simulink library "G2ELib_V1"  (R2020b)
settings: Solver=VariableStepAuto  StartTime=0.0  StopTime=10.0  RelTol=1e-3
undefined symbols (not defined in the file or in its folder): ee_sli_rtmsupport, Filter, Filter_I_ini, Filter_V_ini, gcbh, GFM, GFM_L2, GFM_R2, Parameters_Ib, Parameters_Sb, Parameters_Un_dc, q_filter_wf, References_Q, References_Theta_Eg0, simlt, sps_rtmsupport, Vdc_loop
libraries: powerlib x48, simulink_extras x11, eeTransforms x10, pid_lib x8, spsSourcesModel x3, powerlib_meascontrol x3, spsVIMeasurementModel x3, spsFirstOrderFilterModel x3, spsSynchronousMachineModel x3, eeGeneralControl x2, eePowerMeasurement x1, sps3phSaturableTransformerModel x1
(part 2 of 5)

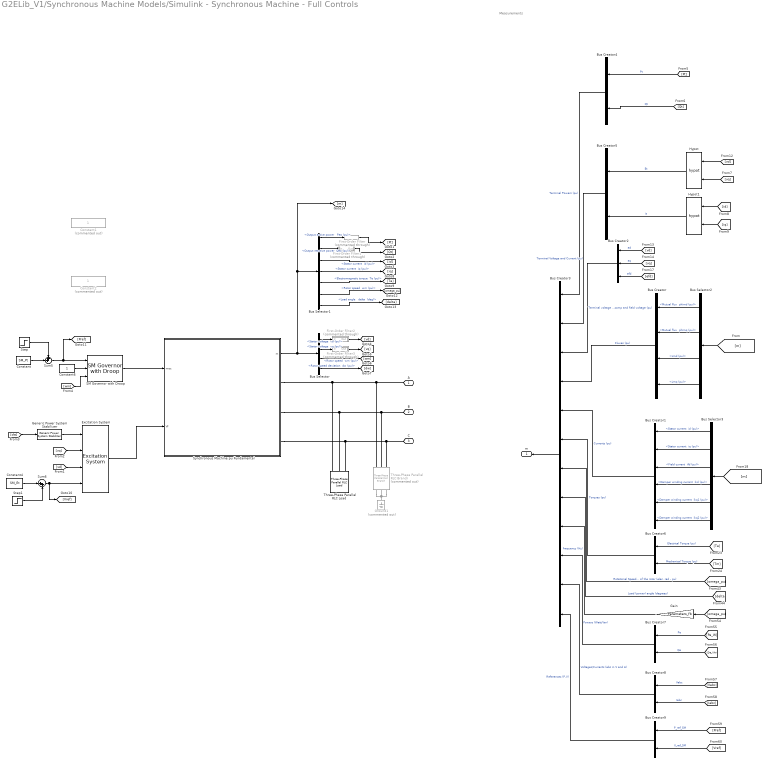
== system G2ELib_V1/Synchronous Machine Models/Simulink - Synchronous Machine - Full Controls ==
  note: Measurements
  Bus Creator : BusCreator  Inputs=4
  Bus Creator1 : BusCreator  Inputs=6
  Bus Creator2 : BusCreator  Inputs=3
  Bus Creator3 : BusCreator  Inputs=12
  Bus Creator{4..9} (6 alike) : BusCreator  Inputs=2
  Bus Selector : BusSelector  OutputSignals="dq0 components.Stator voltage  vd (pu),dq0 components.Stator voltage  vq (pu),Mechanical.Rotor speed  wm (pu),Mechanical.Rotor speed deviation  dw (pu)"
  Bus Selector1 : BusSelector  OutputSignals="Output active power   Peo (pu),Output reactive power  Qeo (pu),dq0 components.Stator current  id (pu),dq0 components.Stator current  iq (pu),Mechanical.Electromagnetic torque  Te (pu),Mechanical.Rotor speed  wm (pu),Load angle   delta  (deg)"
  Bus Selector2 : BusSelector  OutputSignals="dq0 components.Mutual flux  phimd (pu),dq0 components.Mutual flux  phimq (pu),dq0 components.Lmd (pu),dq0 components.Lmq (pu)"
  Bus Selector3 : BusSelector  OutputSignals="dq0 components.Stator current  id (pu),dq0 components.Stator current  iq (pu),dq0 components.Field current  ifd (pu),dq0 components.Damper winding current  ikd (pu),dq0 components.Damper winding current  ikq1 (pu),dq0 components.Damper winding current  ikq2 (pu)"
  Constant : Constant  Value=SM_Pt
  Constant1 : Constant  Commented=on
  Constant2 : Constant  Commented=on
  Constant4 : Constant  Value=SM_Et
  Constant6 : Constant
  Excitation System : sps_avr/Excitation System  tr=SM_Tr  reg=[ SM_Ka, SM_Ta ]  exc=[ SM_Ke, SM_Te ]  tgr=[ SM_Tb, SM_Tc ]  damp=[ SM_Kf, SM_Tf ]  sat=[ 0, 0 ]  lim=[ SM_Efmin, SM_Efmax, SM_Kp ]  v0=[SM_Et 1]
      settings: SourceProductBaseCode=PS
  First-Order Filter : powerlib_meascontrol/Filters/First-Order Filter  Commented=through  FilterType=Lowpass  Tc=20e-3  Ts=0  Initialize=on  Vac_Init=[0, 0, 60]  Vdc_Init=0  PlotResponse=off  FreqRange="[0,  200,  1]"
  First-Order Filter1 : Subsystem  Commented=through  DialogController=POWERSYS.PowerSysDialog  LoadFcn=sps_rtmsupport('LoadFcn', gcbh);  StartFcn=sps_rtmsupport('StartFcn', gcbh);  StopFcn=sps_rtmsupport('StopFcn', gcbh);  mask(First-Order Filter){FilterType=Lowpass, Tc=20e-3, Ts=0, Initialize=on, Vac_Init=[0, 0, 60], Vdc_Init=0, PlotResponse=off, FreqRange=[0,  200,  1]}
      mask prompts: FilterType "Filter type:"; Tc "Time constant (s):"; Ts "Sample time:"; Initialize "Initialize filter states"; Vac_Init "AC initial input [ Mag, Phase (degrees), Freq (Hz) ]:"; Vdc_Init "DC initial input:"; PlotResponse "Plot filter response"; FreqRange "Frequency range (Hz) [Start, End, Inc.]:"
      mask help:
      | Implement a first-order filter.
      |
      | Filter type = Lowpass -> H(s) =  1/(1+T.s)
      | Filter type = Highpass -> H(s) =  T.s/(1+T.s)
      mask init:
      | block=gcb;
      | [WantBlockChoice,Ts,sps] = powericon('FirstOrderFilterInit',block,FilterType,Tc,Initialize,Vac_Init,Vdc_Init,Ts);
      | powericon('FirstOrderFilterInit',FilterType, Tc, PlotResponse, FreqRange);
      | powericon('SetInternalModels','set',block,WantBlockChoice);
      settings: CopyFcn=sps_rtmsupport('CopyFcn', gcbh);  DeleteFcn=sps_rtmsupport('DeleteFcn', gcbh);  UndoDeleteFcn=sps_rtmsupport('UndoDeleteFcn', gcbh);  ModelCloseFcn=sps_rtmsupport('ModelCloseFcn', gcbh);  PreSaveFcn=sps_rtmsupport('PreSaveFcn', gcbh);  PostSaveFcn=sps_rtmsupport('PostSaveFcn', gcbh);  NameChangeFcn=sps_rtmsupport('NameChangeFcn', gcbh);  PreCopyFcn=sps_rtmsupport('PreCopyFcn', gcbh);  OpenFcn="sps_rtmsupport('OpenFcn', gcbh, [1  4  7]);"  CloseFcn=sps_rtmsupport('CloseFcn', gcbh);  PreDeleteFcn=sps_rtmsupport('PreDeleteFcn', gcbh);
      mask Help: helpview(psbhelp);
      mask TypeOptions FilterType: Lowpass | Highpass
      mask Callback Initialize: powericon('FirstOrderFilterInit',gcb);
      mask Callback PlotResponse: powericon('FirstOrderFilterInit',gcb);
      mask Display: plot(sps.X,sps.Y);
  First-Order Filter2 : Subsystem  Commented=through  DialogController=POWERSYS.PowerSysDialog  LoadFcn=sps_rtmsupport('LoadFcn', gcbh);  StartFcn=sps_rtmsupport('StartFcn', gcbh);  StopFcn=sps_rtmsupport('StopFcn', gcbh);  mask(First-Order Filter){FilterType=Lowpass, Tc=20e-3, Ts=0, Initialize=on, Vac_Init=[0, 0, 60], Vdc_Init=0, PlotResponse=off, FreqRange=[0,  200,  1]}
      mask prompts: FilterType "Filter type:"; Tc "Time constant (s):"; Ts "Sample time:"; Initialize "Initialize filter states"; Vac_Init "AC initial input [ Mag, Phase (degrees), Freq (Hz) ]:"; Vdc_Init "DC initial input:"; PlotResponse "Plot filter response"; FreqRange "Frequency range (Hz) [Start, End, Inc.]:"
      mask help:
      | Implement a first-order filter.
      |
      | Filter type = Lowpass -> H(s) =  1/(1+T.s)
      | Filter type = Highpass -> H(s) =  T.s/(1+T.s)
      mask init: same as G2ELib_V1/Synchronous Machine Models/Simulink - Synchronous Machine - Full Controls/First-Order Filter1
      settings: CopyFcn=sps_rtmsupport('CopyFcn', gcbh);  DeleteFcn=sps_rtmsupport('DeleteFcn', gcbh);  UndoDeleteFcn=sps_rtmsupport('UndoDeleteFcn', gcbh);  ModelCloseFcn=sps_rtmsupport('ModelCloseFcn', gcbh);  PreSaveFcn=sps_rtmsupport('PreSaveFcn', gcbh);  PostSaveFcn=sps_rtmsupport('PostSaveFcn', gcbh);  NameChangeFcn=sps_rtmsupport('NameChangeFcn', gcbh);  PreCopyFcn=sps_rtmsupport('PreCopyFcn', gcbh);  OpenFcn="sps_rtmsupport('OpenFcn', gcbh, [1  4  7]);"  CloseFcn=sps_rtmsupport('CloseFcn', gcbh);  PreDeleteFcn=sps_rtmsupport('PreDeleteFcn', gcbh);
      mask Help: helpview(psbhelp);
      mask TypeOptions FilterType: Lowpass | Highpass
      mask Callback Initialize: powericon('FirstOrderFilterInit',gcb);
      mask Callback PlotResponse: powericon('FirstOrderFilterInit',gcb);
      mask Display: plot(sps.X,sps.Y);
  First-Order Filter3 : Subsystem  Commented=through  DialogController=POWERSYS.PowerSysDialog  LoadFcn=sps_rtmsupport('LoadFcn', gcbh);  StartFcn=sps_rtmsupport('StartFcn', gcbh);  StopFcn=sps_rtmsupport('StopFcn', gcbh);  mask(First-Order Filter){FilterType=Lowpass, Tc=20e-3, Ts=0, Initialize=on, Vac_Init=[0, 0, 60], Vdc_Init=0, PlotResponse=off, FreqRange=[0,  200,  1]}
      mask prompts: FilterType "Filter type:"; Tc "Time constant (s):"; Ts "Sample time:"; Initialize "Initialize filter states"; Vac_Init "AC initial input [ Mag, Phase (degrees), Freq (Hz) ]:"; Vdc_Init "DC initial input:"; PlotResponse "Plot filter response"; FreqRange "Frequency range (Hz) [Start, End, Inc.]:"
      mask help:
      | Implement a first-order filter.
      |
      | Filter type = Lowpass -> H(s) =  1/(1+T.s)
      | Filter type = Highpass -> H(s) =  T.s/(1+T.s)
      mask init: same as G2ELib_V1/Synchronous Machine Models/Simulink - Synchronous Machine - Full Controls/First-Order Filter1
      settings: CopyFcn=sps_rtmsupport('CopyFcn', gcbh);  DeleteFcn=sps_rtmsupport('DeleteFcn', gcbh);  UndoDeleteFcn=sps_rtmsupport('UndoDeleteFcn', gcbh);  ModelCloseFcn=sps_rtmsupport('ModelCloseFcn', gcbh);  PreSaveFcn=sps_rtmsupport('PreSaveFcn', gcbh);  PostSaveFcn=sps_rtmsupport('PostSaveFcn', gcbh);  NameChangeFcn=sps_rtmsupport('NameChangeFcn', gcbh);  PreCopyFcn=sps_rtmsupport('PreCopyFcn', gcbh);  OpenFcn="sps_rtmsupport('OpenFcn', gcbh, [1  4  7]);"  CloseFcn=sps_rtmsupport('CloseFcn', gcbh);  PreDeleteFcn=sps_rtmsupport('PreDeleteFcn', gcbh);
      mask Help: helpview(psbhelp);
      mask TypeOptions FilterType: Lowpass | Highpass
      mask Callback Initialize: powericon('FirstOrderFilterInit',gcb);
      mask Callback PlotResponse: powericon('FirstOrderFilterInit',gcb);
      mask Display: plot(sps.X,sps.Y);
  Gain : Gain  Gain=Parameters_fb
  Generic Power System Stabilizer : powerlib/Machines/Generic Power System Stabilizer  Tsensor=SM_T_LP  K=SM_K_PSS  Twashout=SM_T_HP  Tleadlag1=[SM_T1n SM_T1d]  Tleadlag2=[SM_T2n SM_T2d]  VSlimits=[SM_VSmin SM_VSmax]  Vinit=0  Plot_On=off  MagdB_On=on  FreqRange=logspace(-2,2,500)
      settings: SourceProductBaseCode=PS
  Ground1 : powerlib/Elements/Ground  Commented=on  LConnTagsString=a
  Hypot : Math  Operator=hypot  SaturateOnIntegerOverflow=on
  Hypot1 : Math  Operator=hypot  SaturateOnIntegerOverflow=on
  SM Governor with Droop : eeSmGovernor/SM Governor with Droop  droop_percentage=SM_mp  T_G=SM_Tg  pu_throttle0=SM_Pt
      settings: SourceProductBaseCode=PS
  Step : Step  Time=T_Pref  After=delta_Pref  SampleTime=0
  Step1 : Step  Time=T_Vref  After=delta_Vref  SampleTime=0
  Sum5 : Sum  Inputs=++|
  Sum6 : Sum  Inputs=|++
  Synchronous Machine pu Fundamental : Subsystem  DialogController=POWERSYS.PowerSysDialog  LoadFcn=sps_rtmsupport('LoadFcn',gcbh);  StartFcn=sps_rtmsupport('StartFcn',gcbh);  StopFcn=sps_rtmsupport('StopFcn',gcbh);  mask(Synchronous Machine){PresetModel=No, MechanicalLoad=Mechanical power Pm, ShowDetailedParameters=on, RotorType=Round, Units=per unit fundamental parameters, MeasurementBus=off, NominalParameters=[ SM_Sn  SM_Un   Parameters_fb], Stator=[ SM_Ra  SM_Ll  SM_Lad  SM_Laq ], Field=[ SM_Rfd  SM_Lfd], Dampers2=[SM_R1d, SM_L1d, SM_R1q, SM_L1q, SM_R2q, SM_L2q ], Dampers1=[ 0.0284  0.1713  0.00619  0.7252 ], Mechanical=[ SM_H SM_K_D 1], PolePairs=20, InitialConditions=[0 ((SM_theta_0+SM_Phi)*180/pi) SM_It SM_It SM_It ((SM_alpha+SM_Phi)*180/pi) (-120+((SM_alpha+SM_Phi)*180/pi)) (120+((SM_Phi+SM_alpha)*180/pi)) 1], SetSaturation=off, Saturation=[0.6404,0.7127,0.8441,0.9214,0.9956,1.082,1.19,1.316,1.457;0.7,0.7698,0.8872,0.9466,0.9969,1.046,1.1,1.151,1.201], LoadFlowParameters=[1,0,0,0,0], TsPowergui=0, TsBlock=-1, IterativeModel=Trapezoidal non iterative, IterativeDiscreteModel=Trapezoidal non iterative, BusType=PV, Pref=SM_Pt*SM_Sn, Qref=0, Qmin=-inf, Qmax=inf, PLF=0, QLF=0}
      mask prompts: PresetModel "Preset  model:"; MechanicalLoad "Mechanical input:"; ShowDetailedParameters "Show detailed parameters"; RotorType "Rotor type:"; Units "Mask units:"; MeasurementBus "Use signal names to identify bus labels"; NominalParameters "Nominal power, line-to-line voltage and frequency [ Pn(VA)  Vn(Vrms)  fn(Hz) ]:"; Stator "Stator  [ Rs  Ll  Lmd  Lmq  (Lc) ] (pu):"; Field "Field  [ Rf  Llfd ] (pu):"; Dampers2 "Dampers  [ Rkd  Llkd  Rkq1  Llkq1  Rkq2  Llkq2 ] (pu):"; Dampers1 "Dampers  [ Rkd  Llkd  Rkq1  Llkq1 ] (pu):"; Mechanical "Inertia coefficient, friction factor, pole pairs [ H(s)  F(pu)  p() ]:"; PolePairs "Pole pairs p ():"; InitialConditions "Initial conditions [ dw(%)  th(deg)  ia,ib,ic(pu)  pha,phb,phc(deg)  Vf(pu) ]:"; SetSaturation "Simulate saturation"; Saturation "[ ifd; vt] (pu):"; LoadFlowParameters "Load Flow:   [Bus Type, Active Power,  UAB, phase of UAN ]"; TsPowergui "Sample time of powergui block:"; TsBlock "Sample time (-1 for inherited):"; IterativeDiscreteModel "Discrete solver model"; BusType "Generator type:"; Pref "Active power generation P (W):"; Qref "Reactive power generation Q (var):"; Qmin "Minimum reactive power Qmin (var):"; Qmax "Maximum reactive power Qmax (var):"; PLF "Load flow solution:  P_LF (W):"; QLF "Load flow solution:  Q_LF (var):"
      mask help: Implements a 3-phase synchronous machine modelled in the dq rotor reference frame. Stator windings are connected in wye to an internal neutral point.
      mask init:
      | block = gcb;
      | [Ts,SM,WantBlockChoice,X,Y] = powericon('SynchronousMachineInit',block,TsPowergui,TsBlock,MechanicalLoad,Units,RotorType,NominalParameters,Mechanical,PolePairs,InitialConditions,SetSaturation,Saturation,IterativeModel,MeasurementBus,Stator,Field,Dampers1,Dampers2);
      | powericon('SetInternalModels','set',block,WantBlockChoice); sps_rtmsupport('parametereditingmodes',block, [1 2 3 4 5 6 15 20 21 22]); 
      | powericon('ShaftInput',block);
      settings: CopyFcn=sps_rtmsupport('CopyFcn',gcbh); powericon('psbloadfunction',gcb,'gotofrom','UpdateGotoTag');  DeleteFcn=sps_rtmsupport('DeleteFcn',gcbh);  UndoDeleteFcn=sps_rtmsupport('UndoDeleteFcn',gcbh);  ModelCloseFcn=sps_rtmsupport('ModelCloseFcn',gcbh);  PreSaveFcn=sps_rtmsupport('PreSaveFcn',gcbh);  PostSaveFcn=sps_rtmsupport('PostSaveFcn',gcbh);  NameChangeFcn=sps_rtmsupport('NameChangeFcn',gcbh);  PreCopyFcn=sps_rtmsupport('PreCopyFcn',gcbh);  OpenFcn=sps_rtmsupport('OpenFcn',gcbh, [1 2 3 4 5 6 15 20 21 22]);  CloseFcn=sps_rtmsupport('CloseFcn',gcbh);  PreDeleteFcn=sps_rtmsupport('PreDeleteFcn',gcbh);
      mask Help: helpview(psbhelp);
      mask TypeOptions PresetModel: No | 01: 50Hz 400V 8.1kVA 1500RPM | 02: 50Hz 400V 16kVA 1500RPM | 03: 50Hz 400V 31.3kVA 1500RPM | 04: 50Hz 400V 42.5kVA 1500RPM | 05: 50Hz 400V 60kVA 1500RPM | 06: 50Hz 400V 85kVA 1500RPM | 07: 50Hz 400V 250kVA 1500RPM | 08: 50Hz 400V 325kVA 1500RPM | 09: 50Hz 400V 670kVA 1500RPM | 10: 50Hz 400V 910kVA 1500RPM | 11: 50Hz 400V 1320kVA 1500RPM | 12: 50Hz 400V 2000kVA 1500RPM | 13: 60Hz 460V 10.2kVA 1800RPM | 14: 60Hz 460V 20kVA 1800RPM | 15: 60Hz 460V 37.5kVA 1800RPM | 16: 60Hz 460V 52.5kVA 1800RPM | 17: 60Hz 460V 72.5kVA 1800RPM | 18: 60Hz 460V 100kVA 1800RPM | 19: 60Hz 460V 300kVA 1800RPM | 20: 60Hz 460V 406kVA 1800RPM | 21: 60Hz 460V 800kVA 1800RPM | 22: 60Hz 460V 1075kVA 1800RPM | 23: 60Hz 460V 1588kVA 1800RPM | 24: 60Hz 460V 2500kVA 1800RPM
      mask Callback PresetModel: powericon('SynchronousMachineCback',gcb,'per unit fundamental parameters');
      mask TypeOptions MechanicalLoad: Mechanical power Pm | Speed w | Mechanical rotational port
      mask Callback MechanicalLoad: powericon('SynchronousMachineCback',gcb,'per unit fundamental parameters');
      mask Callback ShowDetailedParameters: %powericon('SynchronousMachineCback',gcb,'per unit fundamental parameters');
      mask TypeOptions RotorType: Salient-pole | Round
      mask Callback RotorType: powericon('SynchronousMachineCback',gcb,'per unit fundamental parameters');
      mask TypeOptions Units: per unit fundamental parameters
      mask Callback SetSaturation: powericon('SynchronousMachineCback',gcb,'per unit fundamental parameters');
      mask TypeOptions IterativeModel: Trapezoidal non iterative | Trapezoidal iterative (alg. loop) | Forward Euler
      mask TypeOptions IterativeDiscreteModel: Trapezoidal non iterative | Trapezoidal iterative (alg. loop) | Trapezoidal robust | Backward Euler robust
      mask TypeOptions BusType: swing | PV | PQ
      mask Callback BusType: powericon('SynchronousMachineCback',gcb,'per unit fundamental parameters');
      mask Callback QLF: sps_rtmsupport('parametereditingmodes',gcbh, [1 2 3 4 5 6 15 20 21 22]);
      mask DialogControl Container4 Prompt: Configuration
      mask DialogControl Container9 Prompt: Measurement output
      mask DialogControl Container6 Prompt: Parameters
      mask DialogControl PlotSaturation Prompt: Plot
      mask DialogControl PlotSaturation Callback:
      | Saturation = evalin('base',get_param(gcbh,'Saturation'));
      | figure;plot(Saturation(1,:),Saturation(2,:),'*-');
      | xlabel(['ifd =', mat2str(Saturation(1,:),4)]);
      | ylabel(['vt =', mat2str(Saturation(2,:),4)]);
      mask DialogControl Advanced Prompt: Advanced
      mask DialogControl Note Prompt: Specialized Power Systems can automatically handle the advanced parameters of the block. For more information, see the settings in the 'Preferences' tab of Powergui block.
      mask DialogControl Control3 Prompt: Discrete solver model:
      mask DialogControl Control5 Prompt: This solver model is not recommended.
      mask DialogControl Control6 Prompt: Why?
      mask DialogControl Control6 Callback: web(fullfile(docroot, 'physmod/sps/powersys/ref/synchronousmachine.html#zmw57dd0e55004'))
      mask DialogControl Container7 Prompt: Load Flow
      mask Display:
      | plot(X.p1,Y.p1,X.p2,Y.p2,X.p3,Y.p3,X.p4,Y.p4,X.p5,Y.p5,X.p6,Y.p6,X.p7,Y.p7)
      | color('blue');
      | plot(X.p8,Y.p8)
      | plot(X.p9,Y.p9)
      | port_label('input',1,SM.PortLabel)
  Three-Phase Parallel RLC Branch : powerlib/Elements/Three-Phase Parallel RLC Branch  Commented=on  LConnTagsString=A|B|C  RConnTagsString=A|B|C  BranchType=R  Resistance=1e8  Inductance=1e-3  Capacitance=1e-11  Measurements=None
      settings: SourceProductBaseCode=PS
  Three-Phase Parallel RLC Load : powerlib/Elements/Three-Phase Parallel RLC Load  LConnTagsString=A|B|C  Configuration=Y (grounded)  NominalVoltage=SM_Un  Vabc=[1e3 1e3 1e3]  Vabcp=[1e3 1e3 1e3]  NominalFrequency=Parameters_fb  UnbalancedPower=off  ActivePower=100e3  InductivePower=0  CapacitivePower=0  Pabc=[10e3 9e3 11e3]  QLabc=[100 90 110]  QCabc=[100 90 110]  Pabcp=[10e3 9e3 11e3]  QLabcp=[100 90 110]  QCabcp=[100 90 110]  Measurements=None  LoadType=constant PQ
  A : PMIOPort  Side=Left
  B : PMIOPort  Port=2  Side=Left
  C : PMIOPort  Port=3  Side=Left
  m : Outport
  wires:
  Bus Creator9/1 -> Bus Creator3/12  "References (P,V)"
  [Vref] -> Bus Creator9/2  "V_ref_SM"
  [Pref] -> Bus Creator9/1  "P_ref_SM"
  Sum6/1 -> [Vref], Excitation System/1
  Step1/1 -> Sum6/2
  Constant4/1 -> Sum6/1
  Sum5/1 -> SM Governor with Droop/1, [Pref]
  Step/1 -> Sum5/1
  Constant/1 -> Sum5/2
  Hypot/1 -> Bus Creator5/1  "Et"
  [Qt] -> Bus Creator4/2  "Qt"
  [Pt] -> Bus Creator4/1  "Pt"
  Bus Creator3/1 -> m/1
  [Iabc] -> Bus Creator8/2  "Iabc"
  [Vabc] -> Bus Creator8/1  "Vabc"
  Bus Creator8/1 -> Bus Creator3/11  "Voltages/Currents (abc in V and A)"
  Bus Creator7/1 -> Bus Creator3/10  "Powers (Watt/Var)"
  [Qe_VAr] -> Bus Creator7/2  "Qe"
  [Pe_W] -> Bus Creator7/1  "Pe"
  Gain/1 -> Bus Creator3/9  "frequency (Hz)"
  [omega_pu] -> Gain/1
  [efd] -> Bus Creator2/3  "efd"
  [vq] -> Bus Creator2/2  "eq"
  [vd] -> Bus Creator2/1  "ed"
  [delta] -> Bus Creator3/8  "Load (power) angle (degrees)"
  [omega_pu] -> Bus Creator3/7  "Rotational Speed of the rotor (elec. rad - pu)"
  [Tm] -> Bus Creator6/2  "Mechanical Torque (pu)"
  Bus Creator6/1 -> Bus Creator3/6  "Torques (pu)"
  [Te] -> Bus Creator6/1  "Electrical Torque (pu)"
  Bus Creator1/1 -> Bus Creator3/5  "Currents (pu)"
  Bus Creator/1 -> Bus Creator3/4  "Fluxes (pu)"
  Bus Creator2/1 -> Bus Creator3/3  "Terminal voltage dq-comp and field voltage (pu)"
  Bus Creator5/1 -> Bus Creator3/2  "Terminal Voltage and Current (pu)"
  Bus Creator4/1 -> Bus Creator3/1  "Terminal Powers (pu)"
  [dw] -> Generic Power System Stabilizer/1
  [iq] -> Hypot1/2
  [id] -> Hypot1/1
  Constant6/1 -> SM Governor with Droop/2
  [vd] -> Excitation System/2
  Hypot1/1 -> Bus Creator5/2  "It"
  Bus Selector/1 -> First-Order Filter2/1(In)  "<Stator voltage  vd (pu)>"
  Bus Selector/4 -> [dw]  "<Rotor speed deviation  dw (pu)>"
  Bus Selector/3 -> [wm]  "<Rotor speed  wm (pu)>"
  Bus Selector/2 -> First-Order Filter3/1(In)  "<Stator voltage  vq (pu)>"
  Synchronous Machine pu Fundamental/1(m) -> [m], Bus Selector1/1, Bus Selector/1
  [vq] -> Excitation System/3
  [wm] -> SM Governor with Droop/3
  Bus Selector1/1 -> First-Order Filter/1  "<Output active power   Peo (pu)>"
  Bus Selector1/2 -> First-Order Filter1/1(In)  "<Output reactive power  Qeo (pu)>"
  [vq] -> Hypot/2
  [vd] -> Hypot/1
  Bus Selector1/3 -> [id]  "<Stator current  id (pu)>"
  Bus Selector1/4 -> [iq]  "<Stator current  iq (pu)>"
  Bus Selector1/5 -> [Te]  "<Electromagnetic torque  Te (pu)>"
  Bus Selector1/6 -> [omega_pu]  "<Rotor speed  wm (pu)>"
  Bus Selector1/7 -> [delta]  "<Load angle   delta  (deg)>"
  Generic Power System Stabilizer/1 -> Excitation System/4
  SM Governor with Droop/1 -> Synchronous Machine pu Fundamental/1(mec)
  Excitation System/1 -> Synchronous Machine pu Fundamental/2(Vf)
  First-Order Filter/1 -> [Pt]
  First-Order Filter1/1(Out) -> [Qt]
  First-Order Filter2/1(Out) -> [vd]
  First-Order Filter3/1(Out) -> [vq]
  [m] -> Bus Selector2/1
  Bus Selector2/1 -> Bus Creator/1  "<Mutual flux  phimd (pu)>"
  Bus Selector2/2 -> Bus Creator/2  "<Mutual flux  phimq (pu)>"
  [m] -> Bus Selector3/1
  Bus Selector3/1 -> Bus Creator1/1  "<Stator current  id (pu)>"
  Bus Selector3/2 -> Bus Creator1/2  "<Stator current  iq (pu)>"
  Bus Selector3/3 -> Bus Creator1/3  "<Field current  ifd (pu)>"
  Bus Selector3/4 -> Bus Creator1/4  "<Damper winding current  ikd (pu)>"
  Bus Selector3/5 -> Bus Creator1/5  "<Damper winding current  ikq1 (pu)>"
  Bus Selector3/6 -> Bus Creator1/6  "<Damper winding current  ikq2 (pu)>"
  Bus Selector2/3 -> Bus Creator/3  "<Lmd (pu)>"
  Bus Selector2/4 -> Bus Creator/4  "<Lmq (pu)>"
  connections:
  Synchronous Machine pu Fundamental/RConn1 -- Three-Phase Parallel RLC Branch/LConn1 -- A/RConn1 -- Three-Phase Parallel RLC Load/LConn1
  Synchronous Machine pu Fundamental/RConn2 -- B/RConn1 -- Three-Phase Parallel RLC Branch/LConn2 -- Three-Phase Parallel RLC Load/LConn2
  Synchronous Machine pu Fundamental/RConn3 -- Three-Phase Parallel RLC Load/LConn3 -- Three-Phase Parallel RLC Branch/LConn3 -- C/RConn1
  Ground1/LConn1 -- Three-Phase Parallel RLC Branch/RConn1 -- Three-Phase Parallel RLC Branch/RConn3 -- Three-Phase Parallel RLC Branch/RConn2

== system G2ELib_V1/DC//AC Converters/Voltage Source Converters (VSC)/Grid-Following VSC (GFL) ==
  note: Rename as "GFL_i" when you put in the network where "i" is the index of the GFL unit {1,2,...}
  note: Three phase voltage source for intialization and power flow - TO BE COMMENTED AFTER INITIALIZATION
  note: Proposed scope for GFL units
  Bus Selector2 : BusSelector  OutputSignals=P_GFL,Setpoints.P_set,Q_GFL,Setpoints.Q_Set,V_GFL,f_GFL,Vdc_GFL,Idc_GFL,I_GFL
  GFLi_measurements : Scope  NumInputPorts=7
  Init_GFL_i : Subsystem  DialogController=POWERSYS.PowerSysDialog  LoadFcn=sps_rtmsupport('LoadFcn',gcbh);  StartFcn=sps_rtmsupport('StartFcn',gcbh);  StopFcn=sps_rtmsupport('StopFcn',gcbh);  mask(Three-Phase Source){InternalConnection=Yg, VoltagePhases=off, Voltage=18000, PhaseAngle=2.1921, Voltage_phases=[25e3 25e3 25e3]/sqrt(3), PhaseAngles_phases=[0 -120 +120], Frequency=60, NonIdealSource=off, SpecifyImpedance=off, Resistance=0.8929, Inductance=16.58e-3, ShortCircuitLevel=100e6, BaseVoltage=18000, XRratio=7, BusType=PV, Pref=105000000, Qref=0, Prefabc=[10e3, 10e3, 10e3], Qrefabc=[0, 0, 0], Qmin=-inf, Qmax=inf}
      mask prompts: InternalConnection "Configuration:"; VoltagePhases "Specify internal voltages for each phase"; Voltage "Phase-to-phase voltage (Vrms):"; PhaseAngle "Phase angle of phase A (degrees):"; Voltage_phases "Line-to-neutral voltages [Va Vb Vc] (Vrms)"; PhaseAngles_phases "Phase angle of line-to-neutral voltages [phia phib phic] (deg)"; Frequency "Frequency (Hz):"; NonIdealSource "Internal"; SpecifyImpedance "Specify short-circuit level parameters"; Resistance "Source resistance (Ohms):"; Inductance "Source inductance (H):"; ShortCircuitLevel "3-phase short-circuit level at base voltage(VA):"; BaseVoltage "Base voltage (Vrms ph-ph):"; XRratio "X/R ratio:"; BusType "Generator type:"; Pref "Active power generation P (W)"; Qref "Reactive power generation Q (var)"; Prefabc "Active power generation [Pa Pb Pc] (W)"; Qrefabc "Reactive power generation [Qa Qb Qc] (var)"; Qmin "Minimum reactive power Qmin or [Qamin,Qbmin Qcmin] (var)"; Qmax "Maximum reactive power Qmax or [Qamax,Qbmax Qcmax] (var)"
      mask help: Three-phase voltage source in series with RL branch.
      mask init: same as G2ELib_V1/Miscellaneous Network Elements/Upstream Network
      settings: CopyFcn=sps_rtmsupport('CopyFcn',gcbh); powericon('psbloadfunction',gcb,'goto','UpdateGotoTag');  DeleteFcn=sps_rtmsupport('DeleteFcn',gcbh);  UndoDeleteFcn=sps_rtmsupport('UndoDeleteFcn',gcbh);  ModelCloseFcn=sps_rtmsupport('ModelCloseFcn',gcbh);  PreSaveFcn=sps_rtmsupport('PreSaveFcn',gcbh);  PostSaveFcn=sps_rtmsupport('PostSaveFcn',gcbh);  NameChangeFcn=sps_rtmsupport('NameChangeFcn',gcbh);  PreCopyFcn=sps_rtmsupport('PreCopyFcn',gcbh);  OpenFcn=sps_rtmsupport('OpenFcn',gcbh, [1,2,8,-9,15]);  CloseFcn=sps_rtmsupport('CloseFcn',gcbh);  PreDeleteFcn=sps_rtmsupport('PreDeleteFcn',gcbh);
      mask Help: helpview(psbhelp);
      mask TypeOptions InternalConnection: Y | Yn | Yg
      mask Callback InternalConnection: %powericon('ThreePhaseSourceCback',gcb);
      mask Callback VoltagePhases: powericon('ThreePhaseSourceCback',gcb);
      mask Callback NonIdealSource: powericon('ThreePhaseSourceCback',gcb);
      mask Callback SpecifyImpedance: powericon('ThreePhaseSourceCback',gcb);
      mask TypeOptions BusType: swing | PV | PQ
      mask Callback BusType: powericon('ThreePhaseSourceCback',gcb);
      mask Callback Qmax: sps_rtmsupport('parametereditingmodes',gcbh, [1,2,8,-9,15]);
      mask DialogControl Parameters Prompt: Parameters
      mask DialogControl Container7 Prompt: Source
      mask DialogControl Container6 Prompt: Impedance
      mask DialogControl LoadFlow Prompt: Load Flow
      mask Display:
      | plot(-180,-50,s5,50,s1,s2,s3,s4,[0,9,18,24,29,30,29,24,18,9,0,-9,-18,-24,-29,-30,-29,-24,-18,-9,0]*1.5-45, [30,29,24,18,9,0,-9,-18,-24,-29,-30,-29,-24,-18,-9,0,9,18,24,29,30]*0.8,[-150,-90],[0,0]);
      | plot(g1,g2,g3,g4,g5,g6);
      | plot([1 2 3 4 5 6 7 8 9 10 11 12 13 14 15 16 17 18 19 20 21].*2.5-72, [0,9,18,24,29,30,29,24,18,9,0,-9,-18,-24,-29,-30,-29,-24,-18,-9,0]./3)
  Mux2 : Mux  Inputs=2
  Mux6 : Mux  Inputs=2
  VSC - GFL - Ideal : Subsystem  mask{index_c=1, Parameters_fb=50, Parameters_wb=314.1593, GFL_Un=20000, GFL_Un_dc=32659.8632, GFL_Sn=1000000, GFL_Ib=40.8248, GFL_Ub=16329.9316, GFL_Ub_dc=32659.8632, GFL_Ib_dc=30.6186, GFL_Pref=0.5, GFL_Qref=0.1, GFL_V=1.0024, GFL_Theta_Eg0=0.0023037, GFL_Vdcref=32659.8632, Delta_Pref_GFL=0.1, Tsw_Pref_GFL=1.5, Delta_Qref_GFL=0.1, Tsw_Qref_GFL=2.5, GFL_DC_link_R=500000, GFL_DC_link_C=0.05, GFL_DC_link_Vdc_init=32659.8632, DC_link_Tdc=1e-3, GFL_R1_pu=0.0025, GFL_R2_pu=0.00013325, GFL_L1_pu=0.007854, GFL_L2_pu=0.00048, GFL_C_pu=0.10972, GFL_R1=1, GFL_R2=0.0533, GFL_L1=0.01, GFL_L2=0.00061115, GFL_C=8.731e-07, Controllers=PLL, GFL_Control_PLL=1, GFL_Control_VIM=0, GFL_Control_SU_theta=1, GFL_Control_SU_omega=1, GFL_vdc_Kp=-15999.9979, GFL_vdc_Ki=-2400725.019, GFL_KQ=-33.3333, GFL_Inner_current_loop_Kp=0.0725, GFL_Inner_current_loop_Ki=112.534, GFL_Inner_current_loop_Kffv=1, PLL_Kp=0.38197, PLL_Ki=22.9252, M_pll_0=-0.04362, VIM_wc=15.708, VIM_wc_ini=0, VIM_Iqd_sat=0.25, VIM_Rr_pu=0.0005, VIM_Lr_pu=0.05, VIM_Lm_pu=0.6, VIM_Rr=0.2, VIM_Lr=0.063662, VIM_Lm=0.76394, VIM_Kp=3.1416, VIM_Kd=0.001, VIM_Nd=100, VIM_H=5.04, VIM_J=0.00010213, VIM_D=0.8, VIM_Inertia_ini=0, VIM_Ke_ini=0, VIM_T_sync=0, VIM_f0=50, VIM_w0=1, GFL_Inner_current_loop_Int_ini_d=0.001247, GFL_Inner_current_loop_Int_ini_q=2.5553e-05, GFL_Filter_I_ini=[ 20.3591     -9.66764     -10.6914 ], GFL_Filter_V_ini=[ 16368.6462     -8063.31011     -8305.33605 ], GFL_Line_I_ini=[ 20.3974     -13.5751     -6.82233 ], GFL_Is0_dq0=[ 0.4988    0.010221           0 ], GFL_Eg0_dq0=[ 1.0024  4.3368e-19           0 ], GFL_Ig0_dq0=[ 0.4988    -0.09976           0 ], GFL_Vm0_dq0=[ 1.0036   0.0039431           0 ], M_d_0=-2.0777e-07, M_q_0=-0.00030664, GFL_theta=1.5793}
      mask prompts: index_c "Converter Number"; Parameters_fb "Nominal frequency (Hz)"; Parameters_wb "Nominal rotational frequency (rad/s)"; GFL_Un "Nominal AC voltage - Un (Urms)"; GFL_Un_dc "Nominal DC Voltage (V)"; GFL_Sn "Nominal Complex Power (VA)"; GFL_Ib "Base AC current (A)"; GFL_Ub "Base AC voltage (V)"; GFL_Ub_dc "Base DC voltage (V)"; GFL_Ib_dc "Base DC current (A)"; GFL_Pref "Active Power reference (p.u)"; GFL_Qref "Reactive Power reference (p.u)"; GFL_V "Initial Load Flow AC Voltage (p.u)"; GFL_Theta_Eg0 "Voltage angle (rad)"; GFL_Vdcref "DC voltage reference (V)"; Delta_Pref_GFL "Reference Active Power Steps"; Tsw_Pref_GFL "Time at which these steps take place (s)"; Delta_Qref_GFL "Reference Reactive Power Steps"; Tsw_Qref_GFL "Time at which these steps take place (s)"; GFL_DC_link_R "Parallel Resistance (ohm)"; GFL_DC_link_C "Parallel Capacitance (F)"; GFL_DC_link_Vdc_init "Initial Capacitor Voltage (V)"; DC_link_Tdc "DC-time response (s)"; GFL_R1_pu "F1 - Per unit Resistance"; GFL_R2_pu "F2 - Per unit Resistance"; GFL_L1_pu "F1 - Per unit Inductance"; GFL_L2_pu "F2 - Per unit Inductance"; GFL_C_pu "Per unit Capacitance"; GFL_R1 "F1 - Resistance (ohm)"; GFL_R2 "F2 - Resistance (ohm)"; GFL_L1 "F1 - Inductance (H)"; GFL_L2 "F2 - Inductance (H)"; GFL_C "Capacitance (C)"; Controllers "Select the control model"; GFL_Control_PLL "PLL"; GFL_Control_VIM "VIM"; GFL_Control_SU_theta "SU Theta (1:PLL, 2:VIM)"; GFL_Control_SU_omega "SU Omega (1:PLL, 2:VIM)"; GFL_vdc_Kp "Proportional constant - Kp"; GFL_vdc_Ki "Integral constant - Ki"; GFL_KQ "Integral constant - Ki"; GFL_Inner_current_loop_Kp "Proportional constant - Kp"; GFL_Inner_current_loop_Ki "Integral constant - Ki"; GFL_Inner_current_loop_Kffv "Feed-forward enable"; PLL_Kp "Proportional constant - Kp"; PLL_Ki "Integral constant - Ki"; M_pll_0 "Integral initialization"; VIM_wc "Filter cut-off frequency"; VIM_wc_ini "Filter initialization"; VIM_Iqd_sat "dq-current saturation"; VIM_Rr_pu "Per-unit rotor resistance"; VIM_Lr_pu "Per-unit rotor inductance"; VIM_Lm_pu "Per-unit mutual inductance"; VIM_Rr "Rotor resistance (ohm)"; VIM_Lr "Rotor inductance (H)"; VIM_Lm "Mutual inductance (H)"; VIM_Kp "Virtual Slip propotional action - Kp"; VIM_Kd "Virtual Slip derivative action - Kp"; VIM_Nd "Virtual Slip filter coefficient - Nd"; VIM_H "Inertia Constant (H)"; VIM_J "Equivalent moment of inertia (J)"; VIM_D "Damping (D)"; VIM_Inertia_ini "Inertia TF initialization"; VIM_Ke_ini "Electric Torque TF initialization"; VIM_T_sync "Synchronization Time (s)"; VIM_f0 "Initial rotor position (Hz)"; VIM_w0 "Initial rotor angular speed (rad/s)"; GFL_Inner_current_loop_Int_ini_d "d-axis"; GFL_Inner_current_loop_Int_ini_q "q-axis"; GFL_Filter_I_ini "Filter Current Init."; GFL_Filter_V_ini "Filter Voltage Init."; GFL_Line_I_ini "Line Current Init."; GFL_Is0_dq0 "Filter Current Init. (dq0)"; GFL_Eg0_dq0 "Filter Voltage Init. (dq0)"; GFL_Ig0_dq0 "Line Current Init. (dq0)"; GFL_Vm0_dq0 "Initial Voltage Modulation (dq0)"; M_d_0 "d-axis Vdc controller integrator"; M_q_0 "d-axis Qref controller integrator"; GFL_theta "Initial Phase (rad)"
      mask TypeOptions Controllers: PLL | VIM
      mask DialogControl DescTextVar Prompt: Voltage Source Converter modelled as 3-phase ideal voltage source with cascaded Grid-following/Feeding control topology
      mask DialogControl Container6 Prompt: General Parameters
      mask DialogControl Container9 Prompt: Index
      mask DialogControl Container10 Prompt: Nominal Values
      mask DialogControl Container54 Prompt: Base Values
      mask DialogControl Container12 Prompt: References
      mask DialogControl Container52 Prompt: Events
      mask DialogControl Container7 Prompt: Physical Model
      mask DialogControl Container13 Prompt: DC-Link
      mask DialogControl Container14 Prompt: Filter
      mask DialogControl Container8 Prompt: Control Selection
      mask DialogControl Container20 Prompt: Grid Angle Measurement
      mask DialogControl Container18 Prompt: Synchronization Unit Configuration and Selection
      mask DialogControl Container22 Prompt: Control Parameters
      mask DialogControl Container25 Prompt: Outer Loop Controllers
      mask DialogControl Container23 Prompt: D-axis Vdc Control
      mask DialogControl Container43 Prompt: Q-axis Qref Control
      mask DialogControl Container34 Prompt: Inner Loops
      mask DialogControl Container36 Prompt: Current Loop
      mask DialogControl Container46 Prompt: Grid Angle Measurement
      mask DialogControl Container47 Prompt: PLL
      mask DialogControl Container48 Prompt: VIM
      mask DialogControl Container40 Prompt: Initializations
      mask DialogControl Container41 Prompt: Inner Current Integrators
      mask DialogControl Container51 Prompt: Outer Loop Controls
      mask Display: image('$imagefile'); % Use "Edit Image" on toolstrip to change.
  wires:
  Mux6/1 -> GFLi_measurements/2  "Q_Q_ref"
  Bus Selector2/6 -> GFLi_measurements/4  "<f_GFL>"
  Bus Selector2/1 -> Mux2/1  "<P_GFL>"
  Bus Selector2/4 -> Mux6/2  "<Q_Set>"
  ? -> Bus Selector2/1
  Bus Selector2/8 -> GFLi_measurements/6  "<Idc_GFL>"
  Bus Selector2/5 -> GFLi_measurements/3  "<V_GFL>"
  Bus Selector2/7 -> GFLi_measurements/5  "<Vdc_GFL>"
  Bus Selector2/9 -> GFLi_measurements/7  "<I_GFL>"
  Bus Selector2/2 -> Mux2/2  "<P_set>"
  Mux2/1 -> GFLi_measurements/1  "P_P_ref"
  Bus Selector2/3 -> Mux6/1  "<Q_GFL>"
  VSC - GFL - Ideal/1(m) -> [GFLi_measurements]
  connections:
  Init_GFL_i/RConn1 -- VSC - GFL - Ideal/RConn1
  Init_GFL_i/RConn2 -- VSC - GFL - Ideal/RConn2
  Init_GFL_i/RConn3 -- VSC - GFL - Ideal/RConn3

== system G2ELib_V1/DC//AC Converters/Voltage Source Converters (VSC)/Grid-Forming VSC (GFM) ==
  note: Rename as "GFM_i" when you put in the network where "i" is the index of the GFM unit {1,2,...}
  note: Three phase voltage source for intialization and power flow - TO BE COMMENTED AFTER INITIALIZATION
  note: Proposed scope for GFM units
  Bus Selector13 : BusSelector  OutputSignals=P_GFM,Setpoints.P_set,Q_GFM,Setpoints.Q_set,V_GFM,Setpoints.Eg_set_d,f_GFM,I_GFM,Vdc_GFM,Idc_GFM
  GFMi_measurements : Scope  NumInputPorts=7
  Init_GFM_i : Subsystem  DialogController=POWERSYS.PowerSysDialog  LoadFcn=sps_rtmsupport('LoadFcn',gcbh);  StartFcn=sps_rtmsupport('StartFcn',gcbh);  StopFcn=sps_rtmsupport('StopFcn',gcbh);  mask(Three-Phase Source){InternalConnection=Yg, VoltagePhases=off, Voltage=18000, PhaseAngle=2.1921, Voltage_phases=[25e3 25e3 25e3]/sqrt(3), PhaseAngles_phases=[0 -120 +120], Frequency=60, NonIdealSource=off, SpecifyImpedance=off, Resistance=0.8929, Inductance=16.58e-3, ShortCircuitLevel=100e6, BaseVoltage=18000, XRratio=7, BusType=PV, Pref=105000000, Qref=0, Prefabc=[10e3, 10e3, 10e3], Qrefabc=[0, 0, 0], Qmin=-inf, Qmax=inf}
      mask prompts: InternalConnection "Configuration:"; VoltagePhases "Specify internal voltages for each phase"; Voltage "Phase-to-phase voltage (Vrms):"; PhaseAngle "Phase angle of phase A (degrees):"; Voltage_phases "Line-to-neutral voltages [Va Vb Vc] (Vrms)"; PhaseAngles_phases "Phase angle of line-to-neutral voltages [phia phib phic] (deg)"; Frequency "Frequency (Hz):"; NonIdealSource "Internal"; SpecifyImpedance "Specify short-circuit level parameters"; Resistance "Source resistance (Ohms):"; Inductance "Source inductance (H):"; ShortCircuitLevel "3-phase short-circuit level at base voltage(VA):"; BaseVoltage "Base voltage (Vrms ph-ph):"; XRratio "X/R ratio:"; BusType "Generator type:"; Pref "Active power generation P (W)"; Qref "Reactive power generation Q (var)"; Prefabc "Active power generation [Pa Pb Pc] (W)"; Qrefabc "Reactive power generation [Qa Qb Qc] (var)"; Qmin "Minimum reactive power Qmin or [Qamin,Qbmin Qcmin] (var)"; Qmax "Maximum reactive power Qmax or [Qamax,Qbmax Qcmax] (var)"
      mask help: Three-phase voltage source in series with RL branch.
      mask init: same as G2ELib_V1/Miscellaneous Network Elements/Upstream Network
      settings: CopyFcn=sps_rtmsupport('CopyFcn',gcbh); powericon('psbloadfunction',gcb,'goto','UpdateGotoTag');  DeleteFcn=sps_rtmsupport('DeleteFcn',gcbh);  UndoDeleteFcn=sps_rtmsupport('UndoDeleteFcn',gcbh);  ModelCloseFcn=sps_rtmsupport('ModelCloseFcn',gcbh);  PreSaveFcn=sps_rtmsupport('PreSaveFcn',gcbh);  PostSaveFcn=sps_rtmsupport('PostSaveFcn',gcbh);  NameChangeFcn=sps_rtmsupport('NameChangeFcn',gcbh);  PreCopyFcn=sps_rtmsupport('PreCopyFcn',gcbh);  OpenFcn=sps_rtmsupport('OpenFcn',gcbh, [1,2,8,-9,15]);  CloseFcn=sps_rtmsupport('CloseFcn',gcbh);  PreDeleteFcn=sps_rtmsupport('PreDeleteFcn',gcbh);
      mask Help: helpview(psbhelp);
      mask TypeOptions InternalConnection: Y | Yn | Yg
      mask Callback InternalConnection: %powericon('ThreePhaseSourceCback',gcb);
      mask Callback VoltagePhases: powericon('ThreePhaseSourceCback',gcb);
      mask Callback NonIdealSource: powericon('ThreePhaseSourceCback',gcb);
      mask Callback SpecifyImpedance: powericon('ThreePhaseSourceCback',gcb);
      mask TypeOptions BusType: swing | PV | PQ
      mask Callback BusType: powericon('ThreePhaseSourceCback',gcb);
      mask Callback Qmax: sps_rtmsupport('parametereditingmodes',gcbh, [1,2,8,-9,15]);
      mask DialogControl Parameters Prompt: Parameters
      mask DialogControl Container7 Prompt: Source
      mask DialogControl Container6 Prompt: Impedance
      mask DialogControl LoadFlow Prompt: Load Flow
      mask Display:
      | plot(-180,-50,s5,50,s1,s2,s3,s4,[0,9,18,24,29,30,29,24,18,9,0,-9,-18,-24,-29,-30,-29,-24,-18,-9,0]*1.5-45, [30,29,24,18,9,0,-9,-18,-24,-29,-30,-29,-24,-18,-9,0,9,18,24,29,30]*0.8,[-150,-90],[0,0]);
      | plot(g1,g2,g3,g4,g5,g6);
      | plot([1 2 3 4 5 6 7 8 9 10 11 12 13 14 15 16 17 18 19 20 21].*2.5-72, [0,9,18,24,29,30,29,24,18,9,0,-9,-18,-24,-29,-30,-29,-24,-18,-9,0]./3)
  Mux3 : Mux  Inputs=2
  Mux4 : Mux  Inputs=2
  Mux5 : Mux  Inputs=2
  VSC - GFM - Generic - Ideal : Subsystem  mask{index_c=1, Parameters_fb=50, Parameters_wb=2*pi*50, GFM_Un=20e3, GFM_Un_dc=2*20e3, GFM_Sn=5.22015e+07, GFM_Ib=2610.07662, GFM_Ub=20e3, GFM_Ub_dc=40e3, GFM_Ib_dc=562.5, GFM_Pref=0.5, GFM_Qref=0, GFM_Vref=1, GFM_Theta_Eg0=0, GFM_Vdcref=2*20e3, Delta_Pref_GFM=0, Tsw_Pref_GFM=0, Delta_Vref_GFM=0, Tsw_Vref_GFM=0, DC_link_R=500e6, DC_link_C=0.002, DC_link_Vdc_init=2*20e3, DC_link_Tdc=1e-3, GFM_R1_pu=0.005, GFM_R2_pu=0.15, GFM_L1_pu=0.066, GFM_L2_pu=0.038313, GFM_C_pu=0.066, GFM_R1=0.038313, GFM_R2=0.038313, GFM_L1=0.00365862, GFM_L2=0.00365862, GFM_C=2.741683e-05, Controllers=Droop, Control_PLL=0, Control_VIM=0, Control_MMU_QVDroop=1, Control_MMU_VSM=0, Control_dVOC=0, Control_MMU=1, Control_SU_PfDroop=1, Control_SU_Matching=0, Control_SU_VSM=0, Control_SU_theta=2, Control_SU_omega=2, Control_omega_set=3, Droop_mp=0.02, Droop_nq=0.0001, Droop_wc=0.1*2*pi*50, Droop_Int_ini=0, q_filter_wf=0.1*2*pi*50, q_filter_Int_ini=References_Q, p_filter_Int_ini=0.5, dVOC_eta=1*10/6, dVOC_alpha=12*6/10, Matching_K_theta=0.00005026, VSM_D=1e5, VSM_J=2e3, VSM_AVR_Kp=0.05, VSM_AVR_Ki=11.64, VSM_Dq=100, VSM_K=20, Vdc_loop_Ki=5, Vdc_loop_Kp=0.2, Vdc_loop_Kffi=0, Vdc_loop_Int_ini=2*20e3, Damping_resistor_Enable=1, Damping_resistor_Rv=0.09, Damping_resistor_W_RV=16.66, VI_Enable=0, VI_Rv_pu=0.001, VI_Lv_pu=0.1, TVI_K_RV=0.6716, TVI_Rho_XR=5, TVI_I_thresh_pu=1.2, Inner_voltage_loop_Kp=0.52, Inner_voltage_loop_Ki=1.161022, Inner_voltage_loop_Kffi=1, Inner_current_loop_Kp=0.738891, Inner_current_loop_Ki=1.19, Inner_current_loop_Kffv=1, PLL_Kp=0.4, PLL_Ki=4.69, PLL_Int_ini=0, VIM_wc=0.1*2*pi*50, VIM_wc_ini=0, VIM_Iqd_sat=0.25, VIM_Rr_pu=0.0005, VIM_Lr_pu=0.05, VIM_Lm_pu=0.6, VIM_Rr=0.0048, VIM_Lr=0.0015, VIM_Lm=0.0183, VIM_Kp=3.1416, VIM_Kd=0.001, VIM_Nd=100, VIM_H=0, VIM_J=0.0043, VIM_D=10, VIM_Inertia_ini=0, VIM_Ke_ini=0, VIM_T_sync=0.01, VIM_f0=50.08, VIM_w0=1.0016, SFR_Enable=1, SFR_Rc=0.001, SFR_dP_max=0.1, Inner_voltage_loop_Int_ini_d=0, Inner_voltage_loop_Int_ini_q=0, Inner_current_loop_Int_ini_d=0, Inner_current_loop_Int_ini_q=0, Damping_resistor_Int_ini=0.09, Filter_I_ini=[0 0 0], Filter_V_ini=[0 0 0], Line_I_ini=[0 0 0], Is0_dq0=[0 0 0], Eg0_dq0=[0 0 0], Ig0_dq0=[0 0 0], Vm0_dq0=[0 0 0], dVOC_ini_theta=0, dVOC_ini_R0=[1,0;0,1], Matching_Int_ini=0, GFM_theta=0}
      mask prompts: index_c "Converter Number"; Parameters_fb "Nominal frequency (Hz)"; Parameters_wb "Nominal rotational frequency (rad/s)"; GFM_Un "Nominal AC voltage - Un (Urms)"; GFM_Un_dc "Nominal DC Voltage (V)"; GFM_Sn "Nominal Complex Power (VA)"; GFM_Ib "Base AC current (A)"; GFM_Ub "Base AC voltage (V)"; GFM_Ub_dc "Base DC voltage (V)"; GFM_Ib_dc "Base DC current (A)"; GFM_Pref "Active Power reference (p.u)"; GFM_Qref "Reactive Power reference (p.u)"; GFM_Vref "AC Voltage reference (p.u)"; GFM_Theta_Eg0 "Voltage angle (rad)"; GFM_Vdcref "DC voltage reference (V)"; Delta_Pref_GFM "Reference Active Power Steps"; Tsw_Pref_GFM "Time at which these steps take place (s)"; Delta_Vref_GFM "Reference AC Voltage Steps"; Tsw_Vref_GFM "Time at which these steps take place (s)"; DC_link_R "Parallel Resistance (ohm)"; DC_link_C "Parallel Capacitance (F)"; DC_link_Vdc_init "Initial Capacitor Voltage (V)"; DC_link_Tdc "DC-Response time (s)"; GFM_R1_pu "F1 - Per unit Resistance"; GFM_R2_pu "F2 - Per unit Resistance"; GFM_L1_pu "F1 - Per unit Inductance"; GFM_L2_pu "F2 - Per unit Inductance"; GFM_C_pu "Per unit Capacitance"; GFM_R1 "F1 - Resistance (ohm)"; GFM_R2 "F2 - Resistance (ohm)"; GFM_L1 "F1 - Inductance (H)"; GFM_L2 "F2 - Inductance (H)"; GFM_C "Capacitance (C)"; Controllers "Select the control model"; Control_PLL "PLL"; Control_VIM "VIM"; Control_MMU_QVDroop "MMU - Q-V Droop"; Control_MMU_VSM "MMU - VSM"; Control_dVOC "MMU/SU dVOC"; Control_MMU "MMU (1:QV-droop, 2:dVOC, 3: no MMU,4: VSM AVR)"; Control_SU_PfDroop "SU - P-f Droop"; Control_SU_Matching "SU - Matching"; Control_SU_VSM "SU - VSM"; Control_SU_theta "SU Theta (1:dVOC, 2:Pf-droop, 3:Matching, 4:VSM)"; Control_SU_omega "SU Omega (1:dVOC, 2:Pf-droop, 3:Matching, 4:VSM)"; Control_omega_set "SU Omega Setpoint (1:PLL, 2:VIM, 3: 1 p.u)"; Droop_mp "P-f Droop (mp)"; Droop_nq "Q-V Droop (nq)"; Droop_wc "Second-order Droop filter cut-off frequency"; Droop_Int_ini "Second-order Droop filter initialization"; q_filter_wf "q-filter cut-off frequency"; q_filter_Int_ini "q-filter initialization"; p_filter_Int_ini "p-filter initialization"; dVOC_eta "Eta"; dVOC_alpha "Alpha"; Matching_K_theta "K_theta"; VSM_D "Damping"; VSM_J "Inertia"; VSM_AVR_Kp "AVR - Kp"; VSM_AVR_Ki "AVR - Ki"; VSM_Dq "Q-V proportional constant - Dq"; VSM_K "Q-V integral constant - K"; Vdc_loop_Ki "Integral constant - Ki"; Vdc_loop_Kp "Proportional constant - Kp"; Vdc_loop_Kffi "Feed-forward enable"; Vdc_loop_Int_ini "Integral initialization"; Damping_resistor_Enable "Enable the damping resistor"; Damping_resistor_Rv "Virtual Resistor (Rv)"; Damping_resistor_W_RV "Damping cut-off frequency"; VI_Enable "Enable the VI"; VI_Rv_pu "Virtual Resistor (p.u)"; VI_Lv_pu "Virtual Inductance (p.u)"; TVI_K_RV "TVI Resistor (K_Rv)"; TVI_Rho_XR "TVI R/X ratio (rho)"; TVI_I_thresh_pu "Threshold Current limit (p.u)"; Inner_voltage_loop_Kp "Proportional constant - Kp"; Inner_voltage_loop_Ki "Integral constant - Ki"; Inner_voltage_loop_Kffi "Feed-forward enable"; Inner_current_loop_Kp "Proportional constant - Kp"; Inner_current_loop_Ki "Integral constant - Ki"; Inner_current_loop_Kffv "Feed-forward enable"; PLL_Kp "Proportional constant - Kp"; PLL_Ki "Integral constant - Ki"; PLL_Int_ini "Integral initialization"; VIM_wc "Filter cut-off frequency"; VIM_wc_ini "Filter initialization"; VIM_Iqd_sat "dq-current saturation"; VIM_Rr_pu "Per-unit rotor resistance"; VIM_Lr_pu "Per-unit rotor inductance"; VIM_Lm_pu "Per-unit mutual inductance"; VIM_Rr "Rotor resistance (ohm)"; VIM_Lr "Rotor inductance (H)"; VIM_Lm "Mutual inductance (H)"; VIM_Kp "Virtual Slip propotional action - Kp"; VIM_Kd "Virtual Slip derivative action - Kp"; VIM_Nd "Virtual Slip filter coefficient - Nd"; VIM_H "Inertia Constant (H)"; VIM_J "Equivalent moment of inertia (J)"; VIM_D "Damping (D)"; VIM_Inertia_ini "Inertia TF initialization"; VIM_Ke_ini "Electric Torque TF initialization"; VIM_T_sync "Synchronization Time (s)"; VIM_f0 "Initial rotor position (Hz)"; VIM_w0 "Initial rotor angular speed (rad/s)"; SFR_Enable "Enable/Disable"; SFR_Rc "SFR Constant"; SFR_dP_max "Maximum Regulation (p.u)"; Inner_voltage_loop_Int_ini_d "d-axis"; Inner_voltage_loop_Int_ini_q "q-axis"; Inner_current_loop_Int_ini_d "d-axis"; Inner_current_loop_Int_ini_q "q-axis"; Damping_resistor_Int_ini "Damping resistor integrator"; Filter_I_ini "Filter Current Init."; Filter_V_ini "Filter Voltage Init."; Line_I_ini "Line Current Init."; Is0_dq0 "Filter Current Init. (dq0)"; Eg0_dq0 "Filter Voltage Init. (dq0)"; Ig0_dq0 "Line Current Init. (dq0)"; Vm0_dq0 "Initial Voltage Modulation (dq0)"; dVOC_ini_theta "dVOC Initial Theta"; dVOC_ini_R0 "dVOC R(Kappa) initial"; Matching_Int_ini "Matching integral initialization"; GFM_theta "Initial Phase (rad)"
      mask TypeOptions Controllers: Droop | Droop+PLL | Droop+VIM | dVOC | Matching | VSM
      mask DialogControl Container6 Prompt: General Parameters
      mask DialogControl Container9 Prompt: Index
      mask DialogControl Container10 Prompt: Nominal Values
      mask DialogControl Container54 Prompt: Base Values
      mask DialogControl Container12 Prompt: References
      mask DialogControl Container52 Prompt: Events
      mask DialogControl Container7 Prompt: Physical Model
      mask DialogControl Container13 Prompt: DC-Link
      mask DialogControl Container14 Prompt: Filter
      mask DialogControl Container8 Prompt: Control Selection
      mask DialogControl Container20 Prompt: Grid Angle Measurement
      mask DialogControl Container21 Prompt: Magnitude Modulation Control Configuration and Selection
      mask DialogControl Container18 Prompt: Synchronization Unit Configuration and Selection
      mask DialogControl Container22 Prompt: Control Parameters
      mask DialogControl Container25 Prompt: Outer Loop Controllers
      mask DialogControl Container23 Prompt: GFM-Droop
      mask DialogControl Container24 Prompt: Filters
      mask DialogControl Container43 Prompt: dVOC
      mask DialogControl Container44 Prompt: Matching
      mask DialogControl Container45 Prompt: VSM
      mask DialogControl Container26 Prompt: DC-Side Controller
      mask DialogControl Container27 Prompt: Tertiary Functions
      mask DialogControl Container28 Prompt: Damping Resistor
      mask DialogControl Container31 Prompt: Virtual Impedance (VI)
      mask DialogControl Container33 Prompt: Transient Virtual Impedance (TVI)
      mask DialogControl Container34 Prompt: Inner Loops
      mask DialogControl Container35 Prompt: Voltage Loop
      mask DialogControl Container36 Prompt: Current Loop
      mask DialogControl Container46 Prompt: Grid Angle Measurement
      mask DialogControl Container47 Prompt: PLL
      mask DialogControl Container48 Prompt: VIM
      mask DialogControl Container37 Prompt: Secondary Frequency Regulation
      mask DialogControl Container40 Prompt: Initializations
      mask DialogControl container42 Prompt: Inner Voltage Integrators
      mask DialogControl Container41 Prompt: Inner Current Integrators
      mask DialogControl Container51 Prompt: Outer Loop Controls
      mask Display: image('$imagefile'); % Use "Edit Image" on toolstrip to change.
  wires:
  Bus Selector13/6 -> Mux4/2  "<Eg_set_d>"
  Bus Selector13/9 -> GFMi_measurements/6  "<Vdc_GFM>"
  Bus Selector13/3 -> Mux5/1  "<Q_GFM>"
  Bus Selector13/8 -> GFMi_measurements/5  "<I_GFM>"
  Bus Selector13/10 -> GFMi_measurements/7  "<Idc_GFM>"
  Bus Selector13/2 -> Mux3/2  "<P_set>"
  Mux5/1 -> GFMi_measurements/2  "Q_Q_ref"
  ? -> Bus Selector13/1
  Bus Selector13/1 -> Mux3/1  "<P_GFM>"
  Mux3/1 -> GFMi_measurements/1  "P_P_ref"
  Bus Selector13/7 -> GFMi_measurements/4  "<f_GFM>"
  Bus Selector13/4 -> Mux5/2  "<Q_set>"
  Bus Selector13/5 -> Mux4/1  "<V_GFM>"
  Mux4/1 -> GFMi_measurements/3  "V_V_ref"
  VSC - GFM - Generic - Ideal/1(m) -> [GFMi_measurements]
  connections:
  Init_GFM_i/RConn1 -- VSC - GFM - Generic - Ideal/RConn1
  Init_GFM_i/RConn3 -- VSC - GFM - Generic - Ideal/RConn3
  Init_GFM_i/RConn2 -- VSC - GFM - Generic - Ideal/RConn2

== system G2ELib_V1/Synchronous Machine Models/Simulink - Synchronous Machine - Full Controls/First-Order Filter1 ==
  In : Inport  SampleTime=Ts
  Model : spsFirstOrderFilterModel/Continuous  SystemSampleTime=-1  VariantActivationTime=update diagram  Latency=0  AutoFrameSizeCalculation=off
      settings: SourceProductBaseCode=PS
  Out : Outport  SampleTime=Ts  InitialOutput=0  VectorParamsAs1DForOutWhenUnconnected=off
  wires:
  In/1 -> Model/1
  Model/1 -> Out/1

== system G2ELib_V1/Synchronous Machine Models/Simulink - Synchronous Machine - Full Controls/First-Order Filter2 ==
  In : Inport  SampleTime=Ts
  Model : spsFirstOrderFilterModel/Continuous  SystemSampleTime=-1  VariantActivationTime=update diagram  Latency=0  AutoFrameSizeCalculation=off
      settings: SourceProductBaseCode=PS
  Out : Outport  SampleTime=Ts  InitialOutput=0  VectorParamsAs1DForOutWhenUnconnected=off
  wires:
  Model/1 -> Out/1
  In/1 -> Model/1

== system G2ELib_V1/Synchronous Machine Models/Simulink - Synchronous Machine - Full Controls/First-Order Filter3 ==
  In : Inport  SampleTime=Ts
  Model : spsFirstOrderFilterModel/Continuous  SystemSampleTime=-1  VariantActivationTime=update diagram  Latency=0  AutoFrameSizeCalculation=off
      settings: SourceProductBaseCode=PS
  Out : Outport  SampleTime=Ts  InitialOutput=0  VectorParamsAs1DForOutWhenUnconnected=off
  wires:
  In/1 -> Model/1
  Model/1 -> Out/1
